simulink model "PID"  (R2015a)
settings: Solver=ode45  StartTime=0.0  StopTime=10.0  RelTol=1e-3
settings Model: Creator=HP  LastModifiedBy=HP

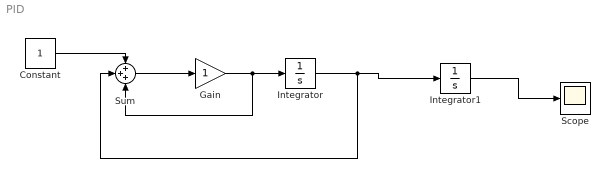
== system PID ==
  Constant : Constant
  Gain : Gain
  Integrator : Integrator
  Integrator1 : Integrator
  Scope : Scope
  Sum : Sum  Inputs=+++
  wires:
  Sum/1 -> Gain/1
  Gain/1 -> Sum/3, Integrator/1
  Integrator1/1 -> Scope/1
  Constant/1 -> Sum/1
  Integrator/1 -> Sum/2, Integrator1/1
